simulink model "vehicle_hostmodel_2022b_Vignesh"  (R2022b)
settings: Solver=VariableStepAuto  StartTime=0  StopTime=1000  RelTol=1e-3
model workspace (MAT data in the model file):
  finalint = 0
  firstWarning = 1
  originalScenarioChecksum = '114339432DE22364D47BB28FC96DC10C'
undefined symbols (not defined in the file): Acceleration, ActorID, AngularVelocity, cameraParams, curvature, DefaultGear, DEND_B, DEND_S, DEND_T, direction, DiscIntNeverNeededParam, driving, gradbp, L, LF, LR, m, matlabshared, MAX_BRAKE, MAX_STEER, MAX_TORQUE, MCAR, MIN_BRAKE, MIN_STEER, MIN_TORQUE, n, NUMD_B, NUMD_S, NUMD_T, Pitch, Pose, Position, psi_o, R, Roll, RRdamp, SceneInfo, sigbuilder_block, STEER_RATIO, stopSign_ID, Tdead, thetaRefs, TL_ID, trackingParams, TrackWidth, Ts, ts, Vdead, Velocity, WB, X_o, xRef2s, Y_o, Yaw, yRef2, yRef2s
libraries: drivingscenarioandsensors x11, simulink x10, roadrunnerscenario x9, slrealtimeutilitieslib x7, slrealtimeiplib x7, simulink_extras x5, drivingvehiclecontroller x3, trackingutilitieslib x3, robotalgslib x2, slpidlib x2, drivinglib x2, eeGeneralControl x1
(part 4 of 5)

== system vehicle_hostmodel_2022b_Vignesh/Reference Data/Subsystem1/Subsystem2/Subsystem ==
  note: Select method to calculate theta
  Integrator : Inport
  Curvature : Lookup_n-D  NumberOfTableDimensions=1  BreakpointsForDimension1=gradbp  Table=curvature  InternalRulePriority=Speed  RndMeth=Simplest
  Direction : Lookup_n-D  NumberOfTableDimensions=1  BreakpointsForDimension1=gradbp  Table=direction  InternalRulePriority=Speed  RndMeth=Simplest
  From Workspace1 : FromWorkspace  VariableName=yRef2  SampleTime=-1
  From Workspace2 : FromWorkspace  VariableName=xRef2  SampleTime=-1
  From Workspace3 : FromWorkspace  VariableName=gradbp  SampleTime=-1
  Goto : Goto  Commented=on  GotoTag=xRef  TagVisibility=global
  Goto1 : Goto  Commented=on  GotoTag=yRef  TagVisibility=global
  Matrix Concatenate : Concatenate  Mode=Multidimensional array  ConcatenateDimension=2
  Mux : Mux  Inputs=3
  Switch Case : SwitchCase
  Theta : Subsystem  Variant=on  VariantControlMode=label  LabelModeActiveChoice=thetaLookUpTable
  X Ref : Lookup_n-D  NumberOfTableDimensions=1  BreakpointsForDimension1=gradbp  Table=xRef2s  InternalRulePriority=Speed  RndMeth=Simplest
  Y Ref : Lookup_n-D  NumberOfTableDimensions=1  BreakpointsForDimension1Source=Input port  BreakpointsForDimension1=gradbp  TableSource=Input port  Table=yRef2s  InternalRulePriority=Speed  RndMeth=Simplest
      settings: InputPortMap=u0,p221,p5
  Out1 : Outport
  Out2 : Outport  Port=2
  CurvatureO : Outport  Port=3
  DirectionO : Outport  Port=4
  finalint : Outport  Port=5
  wires:
  Direction/1 -> DirectionO/1
  Y Ref/1 -> Theta/1(y), Mux/2, Goto1/1
  Theta/1(theta) -> Mux/3
  X Ref/1 -> Theta/2(x), Mux/1, Goto/1
  Matrix Concatenate/1 -> Out1/1
  Curvature/1 -> CurvatureO/1
  Mux/1 -> Out2/1
  From Workspace1/1 -> Y Ref/2, Matrix Concatenate/2
  From Workspace2/1 -> Matrix Concatenate/1
  From Workspace3/1 -> Y Ref/3
  Integrator/1 -> Direction/1, Curvature/1, Theta/3(dis), Y Ref/1, X Ref/1

== system vehicle_hostmodel_2022b_Vignesh/Reference Data/Subsystem1/Subsystem3/Subsystem ==
  note: Select method to calculate theta
  xd : Inport
  yd : Inport  Port=2
  Integrator : Inport  Port=3
  Add Constant : Bias  Bias=6.5  SaturateOnIntegerOverflow=off
  Curvature : Lookup_n-D  NumberOfTableDimensions=1  BreakpointsForDimension1=gradbp  Table=curvature  InternalRulePriority=Speed  RndMeth=Simplest
  Direction : Lookup_n-D  NumberOfTableDimensions=1  BreakpointsForDimension1=gradbp  Table=direction  InternalRulePriority=Speed  RndMeth=Simplest
  From Workspace1 : FromWorkspace  VariableName=yRef2  SampleTime=-1
  From Workspace2 : FromWorkspace  VariableName=xRef2  SampleTime=-1
  From Workspace3 : FromWorkspace  VariableName=gradbp  SampleTime=-1
  Goto : Goto  Commented=on  GotoTag=xRef  TagVisibility=global
  Goto1 : Goto  Commented=on  GotoTag=yRef  TagVisibility=global
  Matrix Concatenate : Concatenate  Mode=Multidimensional array  ConcatenateDimension=2
  Mux : Mux  Inputs=3
  Theta : Subsystem  Variant=on  VariantControlMode=label  LabelModeActiveChoice=thetaLookUpTable
  X Ref : Lookup_n-D  NumberOfTableDimensions=1  BreakpointsForDimension1Source=Input port  BreakpointsForDimension1=gradbp  TableSource=Input port  Table=xRef2s  InternalRulePriority=Speed  RndMeth=Simplest
      settings: InputPortMap=u0,p221,p5
  Y Ref : Lookup_n-D  NumberOfTableDimensions=1  BreakpointsForDimension1Source=Input port  BreakpointsForDimension1=gradbp  TableSource=Input port  Table=yRef2s  InternalRulePriority=Speed  RndMeth=Simplest
      settings: InputPortMap=u0,p221,p5
  Out1 : Outport
  Out2 : Outport  Port=2
  CurvatureO : Outport  Port=3
  DirectionO : Outport  Port=4
  wires:
  Direction/1 -> DirectionO/1
  Theta/1(theta) -> Mux/3
  Matrix Concatenate/1 -> Out1/1
  Curvature/1 -> CurvatureO/1
  Mux/1 -> Out2/1
  From Workspace1/1 -> Add Constant/1, Matrix Concatenate/2
  From Workspace2/1 -> X Ref/2, Matrix Concatenate/1
  From Workspace3/1 -> Y Ref/3, X Ref/3
  X Ref/1 -> Theta/2(x), Mux/1
  Add Constant/1 -> Y Ref/2
  Y Ref/1 -> Theta/1(y), Mux/2
  Integrator/1 -> Direction/1, Curvature/1, Theta/3(dis), Y Ref/1, X Ref/1

== system vehicle_hostmodel_2022b_Vignesh/Reference Data/Subsystem2/Subsystem/Theta ==
  note: 1) Add Subsystem or Model blocks as valid variant choices.
      | 2) You cannot connect blocks at this level. At simulation, connectivity is automatically
      | determined, based on the active variant and port name matching.
  y : Inport
  x : Inport  Port=2
  dis : Inport  Port=3
  thetaBlocks : Subsystem  VariantControl=thetaSimulinkBlock
  thetaLt : Subsystem  VariantControl=thetaLookUpTable
  theta : Outport

== system vehicle_hostmodel_2022b_Vignesh/Reference Data/Subsystem3/Subsystem/Theta ==
  note: 1) Add Subsystem or Model blocks as valid variant choices.
      | 2) You cannot connect blocks at this level. At simulation, connectivity is automatically
      | determined, based on the active variant and port name matching.
  y : Inport
  x : Inport  Port=2
  dis : Inport  Port=3
  thetaBlocks : Subsystem  VariantControl=thetaSimulinkBlock
  thetaLt : Subsystem  VariantControl=thetaLookUpTable
  theta : Outport

== system vehicle_hostmodel_2022b_Vignesh/Roadrunner Port/Initiaal State/Initialize State/Calculate Initial States ==
  EgoRuntime : Inport
  Trigger : TriggerPort  VariantControl=(inherit)  InitialTriggerSignalState=negative  PortDimensions=1
  Calculate Initial States : MATLAB Function  TreatAsAtomicUnit=on
  EgoInitialState : Outport
  wires:
  EgoRuntime/1 -> Calculate Initial States/1(egoRuntime)
  Calculate Initial States/1(egoInitialState) -> EgoInitialState/1

== system vehicle_hostmodel_2022b_Vignesh/Roadrunner Port/Initiaal State/Pack Current States/Delayed Steering System ==
  SteerCmd : Inport
  Add : Sum  Inputs=+-
  Delay : TransferFcn  Denominator=[0.1 0]
  CurrSteer : Outport  VectorParamsAs1DForOutWhenUnconnected=off
  wires:
  Add/1 -> Delay/1
  SteerCmd/1 -> Add/1
  Delay/1 -> CurrSteer/1, Add/2

== system vehicle_hostmodel_2022b_Vignesh/Controllers/Subsystem3/Subsystem1/Subsystem2/Subsystem ==
  acc_cmd : Inport
  Constant1 : Constant  Value=MCAR
  Gain : Gain  Gain=1.1*MCAR
  Gain1 : Gain  Gain=1.2*0.3*2/2
  Gain2 : Gain  Gain=0.7*9.81
  Gain4 : Gain  Gain=R/(7.05*0.8)
  Integrator : Integrator  ExternalReset=falling
  Square : Math  Operator=square
  Sum : Sum  Inputs=+++
  T_eng_cmd : Outport
  wires:
  Constant1/1 -> Gain2/1
  Gain/1 -> Sum/3
  Sum/1 -> Gain4/1
  acc_cmd/1 -> Gain/1, Integrator/2, Integrator/1
  Gain2/1 -> Sum/2
  Gain1/1 -> Sum/1  "F_aero"
  Gain4/1 -> T_eng_cmd/1  "T_eng"
  Integrator/1 -> Square/1  "v"
  Square/1 -> Gain1/1

== system vehicle_hostmodel_2022b_Vignesh/Controllers/Subsystem3/Subsystem1/Subsystem2/Subsystem1 ==
  decc_cmd : Inport
  Constant1 : Constant  Value=MCAR
  Gain : Gain  Gain=1.1*MCAR
  Gain1 : Gain  Gain=1.2*0.3*2/2
  Gain2 : Gain  Gain=0.7*9.81
  Gain4 : Gain  Gain=-R/(7.05*0.8)
  Integrator : Integrator  ExternalReset=falling
  Square : Math  Operator=square
  Sum : Sum  Inputs=+++
  T_brake_cmd : Outport
  wires:
  Square/1 -> Gain1/1
  Integrator/1 -> Square/1  "v"
  Gain4/1 -> T_brake_cmd/1  "T_eng"
  Gain1/1 -> Sum/1  "F_aero"
  Gain2/1 -> Sum/2
  decc_cmd/1 -> Integrator/2, Integrator/1, Gain/1
  Sum/1 -> Gain4/1
  Gain/1 -> Sum/3
  Constant1/1 -> Gain2/1

== system vehicle_hostmodel_2022b_Vignesh/Controllers/Subsystem3/Subsystem2/Subsystem2/Subsystem ==
  acc_cmd : Inport
  Constant1 : Constant  Value=MCAR
  Gain : Gain  Gain=1.1*MCAR
  Gain1 : Gain  Gain=1.2*0.3*2/2
  Gain2 : Gain  Gain=0.7*9.81
  Gain4 : Gain  Gain=R/(7.05*0.8)
  Integrator : Integrator  ExternalReset=falling
  Square : Math  Operator=square
  Sum : Sum  Inputs=+++
  T_eng_cmd : Outport
  wires:
  Constant1/1 -> Gain2/1
  Gain/1 -> Sum/3
  Sum/1 -> Gain4/1
  acc_cmd/1 -> Gain/1, Integrator/2, Integrator/1
  Gain2/1 -> Sum/2
  Gain1/1 -> Sum/1  "F_aero"
  Gain4/1 -> T_eng_cmd/1  "T_eng"
  Integrator/1 -> Square/1  "v"
  Square/1 -> Gain1/1

== system vehicle_hostmodel_2022b_Vignesh/Controllers/Subsystem3/Subsystem2/Subsystem2/Subsystem1 ==
  decc_cmd : Inport
  Constant1 : Constant  Value=MCAR
  Gain : Gain  Gain=1.1*MCAR
  Gain1 : Gain  Gain=1.2*0.3*2/2
  Gain2 : Gain  Gain=0.7*9.81
  Gain4 : Gain  Gain=-R/(7.05*0.8)
  Integrator : Integrator  ExternalReset=falling
  Square : Math  Operator=square
  Sum : Sum  Inputs=+++
  T_brake_cmd : Outport
  wires:
  Square/1 -> Gain1/1
  Integrator/1 -> Square/1  "v"
  Gain4/1 -> T_brake_cmd/1  "T_eng"
  Gain1/1 -> Sum/1  "F_aero"
  Gain2/1 -> Sum/2
  decc_cmd/1 -> Integrator/2, Integrator/1, Gain/1
  Sum/1 -> Gain4/1
  Gain/1 -> Sum/3
  Constant1/1 -> Gain2/1

== system vehicle_hostmodel_2022b_Vignesh/Reference Data/Subsystem1/Subsystem2/Subsystem/Theta ==
  note: 1) Add Subsystem or Model blocks as valid variant choices.
      | 2) You cannot connect blocks at this level. At simulation, connectivity is automatically
      | determined, based on the active variant and port name matching.
  y : Inport
  x : Inport  Port=2
  dis : Inport  Port=3
  thetaBlocks : Subsystem  VariantControl=thetaSimulinkBlock
  thetaLt : Subsystem  VariantControl=thetaLookUpTable
  theta : Outport

== system vehicle_hostmodel_2022b_Vignesh/Reference Data/Subsystem1/Subsystem3/Subsystem/Theta ==
  note: 1) Add Subsystem or Model blocks as valid variant choices.
      | 2) You cannot connect blocks at this level. At simulation, connectivity is automatically
      | determined, based on the active variant and port name matching.
  y : Inport
  x : Inport  Port=2
  dis : Inport  Port=3
  thetaBlocks : Subsystem  VariantControl=thetaSimulinkBlock
  thetaLt : Subsystem  VariantControl=thetaLookUpTable
  theta : Outport

== system vehicle_hostmodel_2022b_Vignesh/Reference Data/Subsystem2/Subsystem/Theta/thetaBlocks ==
  note: theta calculated from Simulink blocks
  y : Inport
  x : Inport  Port=2
  dis : Inport  Port=3
  Atan2 : Trigonometry  Operator=atan2  ApproximationMethod=CORDIC
  Difference : simulink/Discrete/Difference  ICPrevInput=0.0  OutMin=[]  OutMax=[]  OutDataType=fixdt(1, 16)  OutScaling=2^-10  DoSatur=off
  Difference1 : simulink/Discrete/Difference  ICPrevInput=0.0  OutMin=[]  OutMax=[]  OutDataType=fixdt(1, 16)  OutScaling=2^-10  DoSatur=off
  IC : InitialCondition  Value=psi_o
  Radians to Degrees : simulink_extras/Transformations/Radians to Degrees
  Terminator : Terminator
  theta : Outport
  wires:
  IC/1 -> Radians to Degrees/1
  Atan2/1 -> IC/1
  dis/1 -> Terminator/1
  x/1 -> Difference1/1
  y/1 -> Difference/1
  Radians to Degrees/1 -> theta/1
  Difference/1 -> Atan2/1
  Difference1/1 -> Atan2/2

== system vehicle_hostmodel_2022b_Vignesh/Reference Data/Subsystem2/Subsystem/Theta/thetaLt ==
  note: Check out the script "setUpModel" to understand how we have calculated theta
  note: theta based on lookup table
  y : Inport
  x : Inport  Port=2
  dis : Inport  Port=3
  Terminator : Terminator
  Terminator1 : Terminator
  Theta Ref : Lookup_n-D  NumberOfTableDimensions=1  BreakpointsForDimension1=gradbp  Table=thetaRefs  InternalRulePriority=Speed  RndMeth=Simplest
  theta : Outport
  wires:
  Theta Ref/1 -> theta/1
  dis/1 -> Theta Ref/1
  x/1 -> Terminator1/1
  y/1 -> Terminator/1

== system vehicle_hostmodel_2022b_Vignesh/Reference Data/Subsystem3/Subsystem/Theta/thetaBlocks ==
  note: theta calculated from Simulink blocks
  y : Inport
  x : Inport  Port=2
  dis : Inport  Port=3
  Atan2 : Trigonometry  Operator=atan2  ApproximationMethod=CORDIC
  Difference : simulink/Discrete/Difference  ICPrevInput=0.0  OutMin=[]  OutMax=[]  OutDataType=fixdt(1, 16)  OutScaling=2^-10  DoSatur=off
  Difference1 : simulink/Discrete/Difference  ICPrevInput=0.0  OutMin=[]  OutMax=[]  OutDataType=fixdt(1, 16)  OutScaling=2^-10  DoSatur=off
  IC : InitialCondition  Value=psi_o
  Radians to Degrees : simulink_extras/Transformations/Radians to Degrees
  Terminator : Terminator
  theta : Outport
  wires:
  IC/1 -> Radians to Degrees/1
  Atan2/1 -> IC/1
  dis/1 -> Terminator/1
  x/1 -> Difference1/1
  y/1 -> Difference/1
  Radians to Degrees/1 -> theta/1
  Difference/1 -> Atan2/1
  Difference1/1 -> Atan2/2

== system vehicle_hostmodel_2022b_Vignesh/Reference Data/Subsystem3/Subsystem/Theta/thetaLt ==
  note: Check out the script "setUpModel" to understand how we have calculated theta
  note: theta based on lookup table
  y : Inport
  x : Inport  Port=2
  dis : Inport  Port=3
  Terminator : Terminator
  Terminator1 : Terminator
  Theta Ref : Lookup_n-D  NumberOfTableDimensions=1  BreakpointsForDimension1=gradbp  Table=thetaRefs  InternalRulePriority=Speed  RndMeth=Simplest
  theta : Outport
  wires:
  Theta Ref/1 -> theta/1
  dis/1 -> Theta Ref/1
  x/1 -> Terminator1/1
  y/1 -> Terminator/1

== system vehicle_hostmodel_2022b_Vignesh/Reference Data/Subsystem1/Subsystem2/Subsystem/Theta/thetaBlocks ==
  note: theta calculated from Simulink blocks
  y : Inport
  x : Inport  Port=2
  dis : Inport  Port=3
  Atan2 : Trigonometry  Operator=atan2  ApproximationMethod=CORDIC
  Difference : simulink/Discrete/Difference  ICPrevInput=0.0  OutMin=[]  OutMax=[]  OutDataType=fixdt(1, 16)  OutScaling=2^-10  DoSatur=off
  Difference1 : simulink/Discrete/Difference  ICPrevInput=0.0  OutMin=[]  OutMax=[]  OutDataType=fixdt(1, 16)  OutScaling=2^-10  DoSatur=off
  IC : InitialCondition  Value=psi_o
  Radians to Degrees : simulink_extras/Transformations/Radians to Degrees
  Terminator : Terminator
  theta : Outport
  wires:
  IC/1 -> Radians to Degrees/1
  Atan2/1 -> IC/1
  dis/1 -> Terminator/1
  x/1 -> Difference1/1
  y/1 -> Difference/1
  Radians to Degrees/1 -> theta/1
  Difference/1 -> Atan2/1
  Difference1/1 -> Atan2/2

== system vehicle_hostmodel_2022b_Vignesh/Reference Data/Subsystem1/Subsystem2/Subsystem/Theta/thetaLt ==
  note: Check out the script "setUpModel" to understand how we have calculated theta
  note: theta based on lookup table
  y : Inport
  x : Inport  Port=2
  dis : Inport  Port=3
  Terminator : Terminator
  Terminator1 : Terminator
  Theta Ref : Lookup_n-D  NumberOfTableDimensions=1  BreakpointsForDimension1=gradbp  Table=thetaRefs  InternalRulePriority=Speed  RndMeth=Simplest
  theta : Outport
  wires:
  Theta Ref/1 -> theta/1
  dis/1 -> Theta Ref/1
  x/1 -> Terminator1/1
  y/1 -> Terminator/1

== system vehicle_hostmodel_2022b_Vignesh/Reference Data/Subsystem1/Subsystem3/Subsystem/Theta/thetaBlocks ==
  note: theta calculated from Simulink blocks
  y : Inport
  x : Inport  Port=2
  dis : Inport  Port=3
  Atan2 : Trigonometry  Operator=atan2  ApproximationMethod=CORDIC
  Difference : simulink/Discrete/Difference  ICPrevInput=0.0  OutMin=[]  OutMax=[]  OutDataType=fixdt(1, 16)  OutScaling=2^-10  DoSatur=off
  Difference1 : simulink/Discrete/Difference  ICPrevInput=0.0  OutMin=[]  OutMax=[]  OutDataType=fixdt(1, 16)  OutScaling=2^-10  DoSatur=off
  IC : InitialCondition  Value=psi_o
  Radians to Degrees : simulink_extras/Transformations/Radians to Degrees
  Terminator : Terminator
  theta : Outport
  wires:
  IC/1 -> Radians to Degrees/1
  Atan2/1 -> IC/1
  dis/1 -> Terminator/1
  x/1 -> Difference1/1
  y/1 -> Difference/1
  Radians to Degrees/1 -> theta/1
  Difference/1 -> Atan2/1
  Difference1/1 -> Atan2/2

== system vehicle_hostmodel_2022b_Vignesh/Reference Data/Subsystem1/Subsystem3/Subsystem/Theta/thetaLt ==
  note: Check out the script "setUpModel" to understand how we have calculated theta
  note: theta based on lookup table
  y : Inport
  x : Inport  Port=2
  dis : Inport  Port=3
  Terminator : Terminator
  Terminator1 : Terminator
  Theta Ref : Lookup_n-D  NumberOfTableDimensions=1  BreakpointsForDimension1=gradbp  Table=thetaRefs  InternalRulePriority=Speed  RndMeth=Simplest
  theta : Outport
  wires:
  Theta Ref/1 -> theta/1
  dis/1 -> Theta Ref/1
  x/1 -> Terminator1/1
  y/1 -> Terminator/1

== matlab function vehicle_hostmodel_2022b_Vignesh/Environment & Data/Visualisation & Data/Positions and States /MATLAB Function2 ==
  data: Actors input; ss_poses output; ss_State input

function ss_poses = findssposes(Actors, ss_State)

n=length(ss_State);
ss_poses=zeros(n,4);
indices=zeros(n,1);
ID=zeros(length(Actors),1);

for i=1:length(Actors)
 ID(i)=Actors(i).ActorID;
end

indices=find(ismember(ID,ss_State));
if(~isempty(indices))
    
    for i=1:n
        ss_poses(i,:)=([Actors(indices(i)).Position(:)',ss_State(i)]);
    end
end

ss_poses(ss_poses==0)=NaN;






% ss1_poses=zeros(1,4);
% ss2_poses=zeros(1,4);
% for i=1:length(Actors)
%     ID=Actors(i).ActorID;
%     
%     if(ID==ss1_State(1))
%         ss1_poses=[Actors(i).Position(:)',ss1_State(1)];
%     elseif ID== (ss1_State(2))
%         ss2_poses=[Actors(i).Position(:)',ss1_State(2)];
%     
%     end
%   
% end
% ss1_poses(ss1_poses==0)=NaN;   
% ss2_poses(ss2_poses==0)=NaN;

== matlab function vehicle_hostmodel_2022b_Vignesh/Environment & Data/Visualisation & Data/Positions and States /MATLAB Function1 ==
  data: Actors input; TL_poses output; TL_State input

function TL_poses = findTLposes(Actors, TL_State)
n=length(TL_State);
TL_poses=zeros(n/2,5);
indices=zeros(n/2,1);
ID=zeros(length(Actors),1);

for i=1:length(Actors)
 ID(i)=Actors(i).ActorID;
end

indices=find(ismember(ID,TL_State(n/2+1:end)));
if (~isempty(indices))

    for i=1:n/2
        TL_poses(i,:)=([Actors(indices(i)).Position(:)',TL_State(i),ID(indices(i))]);

    end
end
TL_poses(TL_poses==0)=NaN;

== stateflow chart vehicle_hostmodel_2022b_Vignesh/Environment & Data/Visualisation & Data/Positions and States /Traffic Light Sensor/Traffic Light Switching Logic ==
  state STEADYRED
    entry:
    trafficLight(:)= Red; TL_ID=TL_id;
  state STEADYGREEN
    entry:
    trafficLight(:)= Green; TL_ID=TL_id;
  state START
    entry:
    trafficLight=TL_id;
    trafficLight(:)= Black;TL_ID=TL_id;
  state TRAFFICLIGHT_ODDYELLOW_EVENRED
    entry:
    trafficLight(1:2:end)=Yellow;TL_ID(1:2:end)=TL_id(1:2:end);
    trafficLight(2:2:end) = Red;TL_ID(2:2:end)=TL_id(2:2:end);
  state TRAFFICLIGHT_ODDGREEN_EVENRED
    entry:
    trafficLight(1:2:end)=Green;TL_ID(1:2:end)=TL_id(1:2:end);
    trafficLight(2:2:end) = Red;TL_ID(2:2:end)=TL_id(2:2:end);
  state TRAFFICLIGHT_ODDRED_EVENYELLOW
    entry:
    trafficLight(1:2:end)=Red;TL_ID(1:2:end)=TL_id(1:2:end);
    trafficLight(2:2:end) = Yellow;TL_ID(2:2:end)=TL_id(2:2:end);
  state TRAFFICLIGHT_ODDRED_EVENGREEN
    entry:
    trafficLight(1:2:end)=Red;TL_ID(1:2:end)=TL_id(1:2:end);
    trafficLight(2:2:end) = Green;TL_ID(2:2:end)=TL_id(2:2:end);
  (default) -> START
  START -> STEADYGREEN [order 3] : [LightConfig==1]
  START -> STEADYRED [order 1] : [LightConfig==2]
  START -> TRAFFICLIGHT_ODDGREEN_EVENRED [order 2] : [LightConfig ==3]
  TRAFFICLIGHT_ODDGREEN_EVENRED -> TRAFFICLIGHT_ODDYELLOW_EVENRED : after(4,sec)
  TRAFFICLIGHT_ODDYELLOW_EVENRED -> TRAFFICLIGHT_ODDRED_EVENGREEN : after(1,sec)
  TRAFFICLIGHT_ODDRED_EVENYELLOW -> TRAFFICLIGHT_ODDGREEN_EVENRED : after(1,sec)
  TRAFFICLIGHT_ODDRED_EVENGREEN -> TRAFFICLIGHT_ODDRED_EVENYELLOW : after(4,sec)
  data: Green constant double =3; Red constant double =1; Yellow constant double =2; LightConfig input; TL_id input; Black constant double =0; TL_ID output; trafficLight output

== matlab function vehicle_hostmodel_2022b_Vignesh/Environment & Data/Sensors & Perception/MATLAB Function ==
  data: SceneID output; ObjRelVel output; SceneRelVel output; SceneDist output; ObjectDist output; ObjAhead output; SDist input; Tracking input; SceneAhead output; RelVelmin output; RelDistmin output; Trans input; ObjectMIO_Position output
function [SceneID,ObjRelVel,SceneRelVel,SceneDist,ObjectDist,ObjAhead,SceneAhead,RelVelmin,RelDistmin,ObjectMIO_Position]= SFDetections(SDist,Tracking, Trans)
ObjectID = zeros(20,1);
TrackPos = zeros(3,20);
TrackVel = zeros(3,20);
ObjectDist = 100; % zeros(20,1);
SceneDist = 100;
ObjRelVel = 10;
SceneRelVel = 10;
% ScenePos = [0 0];
ObjAhead = 0;
SceneAhead = 0;
SceneID = 0;
TracksNum = Tracking.NumTracks;
ObjectMIO_Position = zeros(3,1);


for t = 1:TracksNum
    ObjectID(t) = Tracking.Tracks(t).ObjectClassID;
    TrackPos(:,t) = Tracking.Tracks(t).State(1:2:5);
    TrackVel(:,t) = Tracking.Tracks(t).State(2:2:6);
   
    if TrackPos(2,t) < 1 && TrackPos(2,t) > -4 && abs(TrackPos(1,t)) <= SDist
        
        if ObjectID(t) >= 7 % 7=SS 8=TL 9=RA 10=RRC % labels {1,2,3,4} => {'TrafficLight','StopSign','RailRoadCrossing','RoundAbout'};
            SceneAhead = 1;
            SceneDist = min(SceneDist,TrackPos(1,t));
            if TrackPos(1,t) <= SceneDist
                % ScenePos = TrackPos(1:2,t)';
                SceneRelVel = TrackVel(1,t);
                SceneID = ObjectID(t);
            end
        end

        if ObjectID(t) < 7 && ObjectID(t) > 0
            ObjAhead = 1;
            ObjectDist = min(ObjectDist,TrackPos(1,t));
            ObjectMIO_Position(:,1) = TrackPos(:,t);

            if TrackPos(1,t) <= ObjectDist
                ObjRelVel = TrackVel(1,t);
                ObjID = ObjectID(t);
            end
        end

    end
    
end

if Trans == 1  % ObjectDist <= SceneDist
    RelVelmin = ObjRelVel;
    RelDistmin = ObjectDist;
else
    RelVelmin = min(SceneRelVel,ObjRelVel);
    RelDistmin = min(SceneDist,ObjectDist);
end

== matlab function vehicle_hostmodel_2022b_Vignesh/Vehicle Dynamics/Info2ActorState/MATLAB Function ==
  data: X input; Position output; Y input; Z input
function Position = fcn(X, Y, Z)

Position = [X Y, Z];

== matlab function vehicle_hostmodel_2022b_Vignesh/Subsystem/PathPlanner/MATLAB Function4 ==
  data: Distance output; output input; CurrentPose input; point output
function [Distance,point] = d2f(output,CurrentPose)



%Distance = norm(output(end,:) - CurrentPose(1:2)');
Distance= output(end,1)- CurrentPose(1);
point=output(end,:);

end

%Distance = sqrt(CurrentPose(1)-output(99,1))^2 + (CurrentPose(2)-output(99,2)^2);
%CurrentPose
%output=zeros(99,2);
%lastPoint = output(end,:);
%dx = lastPoint(1) - x;
%dx= output(end,1)-x;
%dy = output(end,2) - y;
%distance = sqrt(dx^2 + dy^2);

== matlab function vehicle_hostmodel_2022b_Vignesh/Environment & Data/Sensors & Perception/MATLAB Function1 ==
  data: EVpos input; yaw input; SceneID input; SceneInfo input; SDir output; SDist input; D2S output
function [SDir,D2S] = SceneFinder(EVpos,yaw, SceneID, SceneInfo, SDist)
D2S = zeros(10,1);
    % dist = zeros(1,length(SceneLocations));
    for j = 1:length(SceneInfo(:,1))
        distXY = SceneInfo(j,1:2) - EVpos(1:2);
        D2S(j) = norm(distXY);
        
%         if (D2S <= SDist)
%             Scene = SceneInfo(j,3); % labels {1,2,3,4} => {'TrafficLight','StopSign','RailRoadCrossing','RoundAbout'};
%             angl = atan2d(distXY(2),distXY(1));
%             angl = angl - yaw;
% %             rot = [cosd(angl) -sind(angl);sind(angl) cosd(angl)];
% %             distXY = rot*distXY';
% %             angl = atan2d(distXY(2),distXY(1));
%             
%             if angl < 0
%                 angl = angl + 360;
%             end
% 
%             if (angl > 315) || (angl <= 45) 
%                 SDir = "N";
%             elseif (angl > 225) && (angl <= 315)
%                 SDir = "E";
%             elseif (angl > 135) && (angl <= 225)
%                 SDir = "S";
%                 D2S = 1000;
%                 angl = 1000;
%                 Scene = 0;
%             elseif (angl > 45) && (angl <= 135)
%                 SDir = "W";
%             else
%                 SDir = "Error";
%             end
%             break
%         else
%             Scene = 0;
%             SDir = " ";
%             angl = 1000;
%             D2S = 1000;
%         end

    end
[val,indx] = min(D2S);

== matlab function vehicle_hostmodel_2022b_Vignesh/Subsystem/Function-Call Subsystem/MATLAB Function2 ==
  data: EgoPosition input; MIOPos input; curvature input; MIOVel input; V_i input; xd output; yd output; laneL input; laneR input; V_desired input; LCinProgress output
function [xd,yd,LCinProgress] = traj(EgoPosition,MIOPos,curvature,MIOVel, V_i, laneL, laneR, V_desired)
Vx_i =0;Vx_f=0;Vy_i=0;Vy_f=0;Ax_i=0;Ax_f=0;Ay_i=0;Ay_f=0;T_i=0;T_f=0;V_f=0;A_f=0;x_set=0;y_set=0;theta4=0;

P = zeros(6,6);
% xq = zeros(1,size(RefPath,1)); yq = zeros(1,size(RefPath,2));
EgoPosition(1,2)=-EgoPosition(1,2)
x_init= EgoPosition(1,1)+0.5; y_init = EgoPosition(1,2)-0.8;
% xq = RefPath(:,1)'; 
% yq = RefPath(:,2)';
num_foc_t = 98;
V_max= V_desired; ad_n=0; vd_n=MIOVel; wd_n=vd_n*curvature;
lane_width = 3.6 * (laneL-laneR); % +1 if left of current lane and -1 if right of current lane
xd = zeros(num_foc_t+1,1); 
yd = zeros(num_foc_t+1,1);
xf =0; 
yf = 0;

    %xf = [EgoPosition(1,1)+ MIOPos(1) ]; yf = [ EgoPosition(1,2)+ MIOPos(2) + lane_width];  
    xf = [EgoPosition(1,1)+ 40 ]; yf = [ EgoPosition(1,2)+ 1.1*lane_width]; % 80
    V_f = V_max;
    W_f = V_f*curvature;
    A_f = 0;

    %dist2crash = sqrt((x_init-MIOPos(1))^2+(y_init-MIOPos(2))^2);
    %dist2crash = 40;
    %T_f = abs(dist2crash/(MIOVel-V_i));
    T_f = 3;
    P = [1, T_i, T_i^2, T_i^3, T_i^4, T_i^5;
         0, 1, 2*T_i, 3*T_i^2, 4*T_i^3, 5*T_i^4;
         0, 0, 2, 6*T_i, 12*T_i^2, 20*T_i^3;
         1, T_f, T_f^2, T_f^3, T_f^4, T_f^5;
         0, 1, 2*T_f, 3*T_f^2, 4*T_f^3, 5*T_f^4;
         0, 0, 2, 6*T_f, 12*T_f^2, 20*T_f^3];

%     mtang4 = (yq(1,index+2)-yq(1,index+1))/(xq(1,index+2)-xq(1,index+1));

    Vx_i = vd_n*cos(theta4); 
    Vy_i = vd_n*sin(theta4); 
    Ax_i = ad_n*cos(theta4)-vd_n*sin(theta4)*wd_n; 
    Ay_i = ad_n*sin(theta4)+vd_n*cos(theta4)*wd_n;

%     if(xq(index+2)-xq(index+1)<0)
%         theta_4 = pi + atan(mtang4);
%     else
%         theta_4 = atan(mtang4);
%     end

    theta_4 =0;
    Vx_f = V_f*cos(theta_4); % curvature angle
    Vy_f = V_f*sin(theta_4);
    Ax_f = A_f*cos(theta_4)-V_f*sin(theta_4)*W_f;
    Ay_f = A_f*sin(theta_4)+V_f*cos(theta_4)*W_f;

    g1 = [x_init; Vx_i; Ax_i; xf; Vx_f; Ax_f];
    g2 = [y_init; Vy_i; Ay_i; yf; Vy_f; Ay_f];

    a_coeff = P\g1;
    b_coeff = P\g2;
    
    td = T_i;
    scatter(x_init,y_init,'go')
    hold on; 
    scatter(xf,yf,'ro')
    hold on;
    
    for f = 1:(num_foc_t+1)
        xd(f,1) = [1,td,td^2,td^3,td^4,td^5]*a_coeff 
        yd(f,1) = [1,td,td^2,td^3,td^4,td^5]*b_coeff
        td = td + (T_f - T_i)/num_foc_t;
        scatter(xd(f,1),yd(f,1),'y.');
    end

LCinProgress = 1;

% hold on;
end

== matlab function vehicle_hostmodel_2022b_Vignesh/Roadrunner Port/Initiaal State/Initialize State/Calculate Initial States/Calculate Initial States ==
  data: egoRuntime input; egoInitialState output Bus: BusVehicleInfo
function egoInitialState = getInitialState(egoRuntime)
%getInitialState calculates initial conditions of the vehicle

% Calculate velocity
velocity = norm(egoRuntime.ActorRuntime.Velocity,2);
% Get Transformation matrix
transformationMatrix = egoRuntime.ActorRuntime.Pose;
% Get pose information
x = transformationMatrix(1,4);
y = transformationMatrix(2,4);
yaw = atan2d(-transformationMatrix(1,2), ...
            transformationMatrix(1,1));
% Pack the initial states
egoInitialState = struct('CurrPose', [y, -x, yaw], ...
    'CurrVelocity', velocity, ...
    'CurrYawRate', 0, ...
    'CurrSteer',0, ...
    'Direction',1);

== matlab function vehicle_hostmodel_2022b_Vignesh/Controllers/Subsystem3/Subsystem2/MATLAB Function ==
  data: u input; accel output; decel output
function [accel, decel] = fcn(u)
if(u>0)
    accel=u; decel=0;
elseif(u<0)
    accel=0; decel=-u;
else
    accel=0;decel=0;
end

== matlab function vehicle_hostmodel_2022b_Vignesh/Controllers/MATLAB Function2 ==
  data: v input; RefVelCmd output; curvature input
function RefVelCmd = fcn(v,curvature)

    if abs(curvature) >= 0 && abs(curvature) <= 1e-2
        RefVelCmd = v;
    else
        r = 1/abs(curvature);
        RefVelCmd = min(v,sqrt(9.81*r*.2));
    end

== matlab function vehicle_hostmodel_2022b_Vignesh/Vehicle Dynamics/Info2ActorState/MATLAB Function1 ==
  data: Xdot input; Velocity output; Ydot input; Zdot input
function Velocity = fcn(Xdot, Ydot, Zdot)

Velocity = [Xdot Ydot, Zdot];

== matlab function vehicle_hostmodel_2022b_Vignesh/Roadrunner Port/MATLAB Function ==
  data: ActorsIn input; EgoVeh input; EgoRefActors output Bus: BusWorldToVehicleActors
function EgoRefActors  = GlobaltoEgoRefConv(ActorsIn,EgoVeh)
%ActorsOut = Simulink.Bus;
ActorsOut = ActorsIn;
numActors = length(ActorsIn.Actors);
for k = 1:numActors
    actorOut = driving.scenario.targetsToEgo(ActorsIn.Actors(k),EgoVeh);
    ActorsOut.Actors(k).ActorID             = actorOut.ActorID;
    ActorsOut.Actors(k).Position            = actorOut.Position;
    ActorsOut.Actors(k).Velocity            = actorOut.Velocity;
    ActorsOut.Actors(k).Roll                = actorOut.Roll;
    ActorsOut.Actors(k).Pitch               = actorOut.Pitch;
    ActorsOut.Actors(k).Yaw                 = actorOut.Yaw;
    ActorsOut.Actors(k).AngularVelocity    = actorOut.AngularVelocity;
end
EgoRefActors = ActorsOut;
end

== matlab function vehicle_hostmodel_2022b_Vignesh/MATLAB Function ==
  data: ttc output; dist output; left output; right output; LL_avail output; RL_avail output; tend2stay output; ego input; act input; LaneBounds input; RoadSpeed input; ego_vel output; stay output; LL_Change output; RL_Change output; y_lane output; LCinProgress input
function [ttc,dist,left,right,LL_avail,RL_avail,tend2stay,ego_vel,stay,LL_Change,RL_Change,y_lane] = fcn(ego,act,LaneBounds,RoadSpeed, LCinProgress)                       


%% Major tasks to look into

% Check the performance while transitioning into another lane 
% Lane change output when the ego on extreme lanes.
% Develop code to handle lane changes on road curvatures
% Integrate with the trajectory generation and check the perfomance
% Convert the code to ego vehicle coordinates


%%
%define some parameters
r_c = 20; %range considered to MIOs
t_min =  2;

num_actors = length(act.Actors);
%num_lanes = length(LaneBounds.LaneBoundaries)-1;


%% Using sensor data 
% TracksNum = Tracking.NumTracks;
% 
% 
% for t = 1:TracksNum
%     ObjectID(t) = Tracking.Tracks(t).ObjectClassID;
%     TrackPos(:,t) = Tracking.Tracks(t).State(1:2:5);
%     TrackVel(:,t) = Tracking.Tracks(t).State(2:2:6);

%% ego position and  velocity magnitude
ego_pos = ego.Position;
ego_vel = ego.Velocity(1);  % velocity

%ttc: (array) : agent.relative position / abs(relative velocity)
ttc = zeros(1,num_actors);
left = zeros(1,num_actors);
right = zeros(1,num_actors);

dist =  zeros(1,num_actors);
tend2stay=1;

%%
y_lane = zeros(1,length(LaneBounds.LaneBoundaries))

for l=1:length(y_lane)
    y_lane(l)=LaneBounds.LaneBoundaries(l).Coordinates(end,2)
end

%%
for i= 1:num_actors

    % Grab actor positions and velocities
    actor_pos = act.Actors(i).Position;   
    actor_vel = act.Actors(i).Velocity(1);  % x-component velocity

    %relative velocity of the agent
    rel_vel = actor_vel - ego_vel;


    %% Check if the actor is within a r_c range. If it is out of range, pass lane change as '1' automatically.

   dist(i) = norm([actor_pos(1) actor_pos(2)]-[ego_pos(1) ego_pos(2)]);
        
    if dist(i) > r_c
        left(i)=1;
        right(i)=1;
        continue
    end

    %% Check if the actor is in the same lane as that of ego

    % If the actor and ego are in the same lane, it is considered a lead/following vehicle in the same lane and by defualt, the lane change flag is 1.

    if (actor_pos(2)< (ego_pos(2)+0.5) && actor_pos(2) > (ego_pos(2)-0.5))
        if (rel_vel < 0 && ego_vel < (RoadSpeed+5) && actor_pos(1) > ego_pos(1) )
            left(i) =1;
            right(i)=1;
            tend2stay=0;        % we need to incorporate too slow condition even when the relative velocity is greater than 0.

        elseif (rel_vel < 0 && ego_vel < (RoadSpeed+5) && actor_pos(1) < ego_pos(1) )
            left(i) =1;
            right(i)=1;
            tend2stay=1;
        end

        continue
    end

    
    %% calculate ttc for the rest of the vehicles


    ttc(i) = (actor_pos(1)-ego_pos(1))/abs(rel_vel);

    % checking conditions for other surrounding actors

    % all actors on the left lane of the ego vehicle
%%
    if actor_pos(2)-ego_pos(2) > 0  

        if and(rel_vel>0, ttc(i) > t_min)  % target vehicles on the front of ego vehicle (any lane)
    
            left(i)=1; 
            right(i)=1;
    
        elseif (ttc(i)<0 && rel_vel<0 && abs(ttc(i)) > t_min)    % target vehicle on the back of ego vehicle (ttc<0) (any lane)
            left(i) =1;
            right(i)=1;
    
        else 
            left(i) =0;
            right(i)=1;
    
        end

    % all actors on the right lane of the ego vehicle

    elseif actor_pos(2)-ego_pos(2) < 0
         
        if and(rel_vel>0, ttc(i) > t_min)  % target vehicles on the front of ego vehicle (any lane)
    
            left(i)=1;
            right(i)=1;
    
        elseif (ttc(i)<0 && rel_vel<0 && abs(ttc(i)) > t_min)    % target vehicle on the back of ego vehicle (ttc<0) (any lane)
            left(i) =1;
            right(i)=1;
    
        else 
            left(i) =1;
            right(i)=0;
    
        end
    end
%%

end

%% check if the vehicle is in the extreme end lanes

    if ego_pos(2)<y_lane(1) && ego_pos(2)>y_lane(2)

        LL=0; RL=1;
    elseif ego_pos(2) > y_lane(end) && ego_pos(2) < y_lane(end-1)
        RL=0; LL=1;
    else 

        RL=1;LL=1;
    end

%%
LL_avail = all(left) %&& LL;

RL_avail = all(right) %&& RL               %&& ~lcLeft ; this can be decided later 


%% final commands

stay = tend2stay || ~(tend2stay || LL_avail || RL_avail);
LL_Change =  ~tend2stay && LL_avail ;

RL_Change =  ~tend2stay && RL_avail && ~LL_Change ;
LCFlag = ~stay;
if LCFlag && LCinProgress
    LCFlag = false;
    stay = ~LCFlag;
end

%% 






end

== matlab function vehicle_hostmodel_2022b_Vignesh/Vehicle Dynamics/Info2ActorState/MATLAB Function2 ==
  data: aX input; Acceleration output; aY input; aZ input
function Acceleration = fcn(aX, aY, aZ)

Acceleration = [aX aY, aZ];

== matlab function vehicle_hostmodel_2022b_Vignesh/Vehicle Dynamics/Info2ActorState/MATLAB Function3 ==
  data: phiDot input; AngularVelocity output; thetaDot input; psiDot input
function AngularVelocity = fcn(phiDot, thetaDot, psiDot)

AngularVelocity = [phiDot thetaDot, psiDot];

== stateflow chart vehicle_hostmodel_2022b_Vignesh/Vehicle Dynamics/VehicleDynamics/engine-steer-brake dynamics/GearSelection1 ==
  state Park
    CurrGear = 0;
  state Reverse
    CurrGear = -1;
  state drive
    CurrGear = 1;
  (default) -> (junction 12)
  (junction 12) -> Reverse [order 3] : [DefaultGear == -1]
  (junction 12) -> drive [order 2] : [DefaultGear == 1]
  (junction 12) -> Park [order 1] : [DefaultGear == 0]
  (junction 12) -> Park [order 4] : %fallback to park
  drive -> Park [order 2] : [gear_cmd == 0 && allowShift(vc,Tbrake)]
  Park -> Reverse [order 2] : [gear_cmd == -1 && allowShift(vc,Tbrake)]
  Park -> drive [order 1] : [gear_cmd == 1 && allowShift(vc,Tbrake)]
  Reverse -> Park [order 2] : [gear_cmd == 0 && allowShift(vc,Tbrake)]
  drive -> Reverse [order 1] : [gear_cmd == -1 && allowShift(vc,Tbrake)]
  Reverse -> drive [order 1] : [gear_cmd == 1 && allowShift(vc,Tbrake)]
  data: Tdead parameter; Vdead parameter; vel function_input; brakeT function_input; allow function_output; CurrGear output; Tbrake input; vc input; gear_cmd input; DefaultGear parameter
  function allow = allowShift(vel, brakeT):
    | function allow = allowShift(vel, brakeT)
    | allow = (abs(vel) <= Vdead) && (abs(brakeT)>Tdead);
    | end

== matlab function vehicle_hostmodel_2022b_Vignesh/Vehicle Dynamics/VehicleDynamics/engine-steer-brake dynamics/compute net torque ==
  data: gear input; Tnet output; Tengine input; Tbrake input; vc input
function Tnet  = net_torque(gear,Tengine,Tbrake,vc)

%  --set engine torque based on current gear selection

if (gear == 0)
    %  --vehicle is in PARK, so force engine torque to zero
    Tengine = 0;
end

Tnet = Tengine + Tbrake*tanh(5*vc);

end

== matlab function vehicle_hostmodel_2022b_Vignesh/Vehicle Dynamics/VehicleDynamics/engine-steer-brake dynamics/gear selection state machine ==
  data: gear output; gear_cmd input; vc input; Tbrake input; Tdead input; Vdead input
function gear = gear_change_FSM(gear_cmd,vc,Tbrake,Tdead,Vdead)

persistent GEAR

%  The vehicle gear can take on one of the following enumerated values:
%  -1 = REVERSE
%   0 = PARK
%   1 = DRIVE

%  --initialize the local persistent variables

if isempty(GEAR)
    %  --default gear at startup is PARK
    %  Note:  Change this to 1 if you want car to initialize in DRIVE
    GEAR = 0;
end


%  --evaluate the gear change finite state machine

switch GEAR
    case 0  % vehicle is in PARK
        if (gear_cmd == 1)
            %  --check to see if we can shift to DRIVE
            if ((abs(vc) <= Vdead) && (abs(Tbrake) > Tdead))
                %  --shift to DRIVE
                GEAR = 1;
            end
            
        elseif (gear_cmd == 2)
            %  --check to see if we can shift to REVERSE
            if ((abs(vc) <= Vdead) && (abs(Tbrake) > Tdead))
                %  --shift to REVERSE
                GEAR = 2;
            end
        end
        
    case 1  % vehicle is in DRIVE
        if (gear_cmd == 0)
            %  --check to see if we can shift to PARK
            if ((abs(vc) <= Vdead) && (abs(Tbrake) > Tdead))
                %  --shift to PARK
                GEAR = 0;
            end
            
        elseif (gear_cmd == 2)
            %  --check to see if we can shift to REVERSE
            if ((abs(vc) <= Vdead) && (abs(Tbrake) > Tdead))
                %  --shift to REVERSE
                GEAR = 2;
            end
        end
        
    case -1  % vehicle is in REVERSE
        if (gear_cmd == 0)
            %  --check to see if we can shift to PARK
            if ((abs(vc) <= Vdead) && (abs(Tbrake) > Tdead))
                %  --shift to PARK
                GEAR = 0;
            end
            
        elseif (gear_cmd == 1)
            %  --check to see if we can shift to DRIVE
            if ((abs(vc) <= Vdead) && (abs(Tbrake) > Tdead))
                %  --shift to DRIVE
                GEAR = 1;
            end
        end
        
    otherwise  %  --should never be here
        if (vc > Vdead)
            %  --moving forward, so must be in DRIVE
            GEAR = 1;
        elseif (vc < -Vdead)
            %  --moving backward, so must be in REVERSE
            GEAR = 2;
        else
            %  --vehicle stoppped, so must be in PARK
            GEAR = 0;
        end

end


%  --output the current actual gear setting

gear = GEAR;

return

== matlab function vehicle_hostmodel_2022b_Vignesh/Controllers/Lateral Controllers1/Swicth 1 ==
  data: stan input; y output; pure input
function y = fcn(stan, pure)

if stan<pure
    y=stan
else
    y=pure
end

== matlab function vehicle_hostmodel_2022b_Vignesh/Roadrunner Port/Pack Actor Pose/Pose Generation ==
  data: pose input; currPose output
function currPose = generatePose(pose)

yaw = deg2rad(pose(3));
rotm = eul2rotm([yaw 0 0]);

currPose = [[rotm [pose(1:2) 0]']; [0 0 0 1]];

== matlab function vehicle_hostmodel_2022b_Vignesh/Controllers/Lateral Controllers1/Average ==
  data: stan input; y output; pure input
function y = fcn(stan, pure)

y=(stan+pure)/2

== matlab function vehicle_hostmodel_2022b_Vignesh/Subsystem/Function-Call Subsystem/MATLAB Function1 ==
  data: EgoPosition input; MIOPos input; curvature input; MIOVel input; V_i input; xd output; yd output; laneL input; laneR input; V_desired input; LCinProgress output
function [xd,yd,LCinProgress] = traj(EgoPosition,MIOPos,curvature,MIOVel, V_i, laneL, laneR, V_desired)
Vx_i =0;Vx_f=0;Vy_i=0;Vy_f=0;Ax_i=0;Ax_f=0;Ay_i=0;Ay_f=0;T_i=0;T_f=0;V_f=0;A_f=0;x_set=0;y_set=0;theta4=0;

P = zeros(6,6);
% xq = zeros(1,size(RefPath,1)); yq = zeros(1,size(RefPath,2));
EgoPosition(1,2)=-EgoPosition(1,2);
x_init= EgoPosition(1,1)+2; y_init = EgoPosition(1,2)-2;
% xq = RefPath(:,1)'; 
% yq = RefPath(:,2)';
num_foc_t = 98;
V_max= V_desired; ad_n=0; vd_n=MIOVel; wd_n=vd_n*curvature;
lane_width = 3.6 * (laneL-laneR); % +1 if left of current lane and -1 if right of current lane(rahul flipped)
xd = zeros(num_foc_t+1,1); 
yd = zeros(num_foc_t+1,1);
xf =0; 
yf = 0;

    %xf = [EgoPosition(1,1)+ MIOPos(1) ]; yf = [ EgoPosition(1,2)+ MIOPos(2) + lane_width];  
    xf = [EgoPosition(1,1)+ 20 ]; yf = [EgoPosition(1,2)+ lane_width]; % 80
    V_f = V_max;
    W_f = V_f*curvature;
    A_f = 0;

    %dist2crash = sqrt((x_init-MIOPos(1))^2+(y_init-MIOPos(2))^2);
    %dist2crash = 40;
    %T_f = abs(dist2crash/(MIOVel-V_i));
    T_f = 3;
    P = [1, T_i, T_i^2, T_i^3, T_i^4, T_i^5;
         0, 1, 2*T_i, 3*T_i^2, 4*T_i^3, 5*T_i^4;
         0, 0, 2, 6*T_i, 12*T_i^2, 20*T_i^3;
         1, T_f, T_f^2, T_f^3, T_f^4, T_f^5;
         0, 1, 2*T_f, 3*T_f^2, 4*T_f^3, 5*T_f^4;
         0, 0, 2, 6*T_f, 12*T_f^2, 20*T_f^3];

%     mtang4 = (yq(1,index+2)-yq(1,index+1))/(xq(1,index+2)-xq(1,index+1));

    Vx_i = vd_n*cos(theta4); 
    Vy_i = vd_n*sin(theta4); 
    Ax_i = ad_n*cos(theta4)-vd_n*sin(theta4)*wd_n; 
    Ay_i = ad_n*sin(theta4)+vd_n*cos(theta4)*wd_n;

%     if(xq(index+2)-xq(index+1)<0)
%         theta_4 = pi + atan(mtang4);
%     else
%         theta_4 = atan(mtang4);
%     end

    theta_4 =0;
    Vx_f = V_f*cos(theta_4); % curvature angle
    Vy_f = V_f*sin(theta_4);
    Ax_f = A_f*cos(theta_4)-V_f*sin(theta_4)*W_f;
    Ay_f = A_f*sin(theta_4)+V_f*cos(theta_4)*W_f;

    g1 = [x_init; Vx_i; Ax_i; xf; Vx_f; Ax_f];
    g2 = [y_init; Vy_i; Ay_i; yf; Vy_f; Ay_f];

    a_coeff = P\g1;
    b_coeff = P\g2;
    
    td = T_i;
    scatter(x_init,y_init,'go')
    hold on; 
    scatter(xf,yf,'ro')
    hold on;
    
    for f = 1:(num_foc_t+1)
        xd(f,1) = [1,td,td^2,td^3,td^4,td^5]*a_coeff 
        yd(f,1) = [1,td,td^2,td^3,td^4,td^5]*b_coeff
        td = td + (T_f - T_i)/num_foc_t;
        scatter(xd(f,1),yd(f,1),'y.');
    end

LCinProgress = 1;

% hold on;
end

== matlab function vehicle_hostmodel_2022b_Vignesh/Roadrunner Port/Pack Actor Pose/Velocity XYZ Components ==
  data: yaw input size=1; velocity output size=[1 3]; speed input size=1
function velocity = computeVelocity(yaw, speed)

% Output velocity vector (x,y,z)
velocity = speed * [-sind(yaw) cosd(yaw) 0];

== matlab function vehicle_hostmodel_2022b_Vignesh/Roadrunner Port/ENU to NWD/MATLAB Function ==
  data: traj input; destination_traj output; last_idx output
function [destination_traj,last_idx] = DestinationPoint(traj)

last_idx = 1;

for i=1:length(traj)
    if norm(traj(i,1:2)) == 0
        last_idx = i-1;
        break
    end
end

destination_traj = traj(last_idx,1:2);

end

== matlab function vehicle_hostmodel_2022b_Vignesh/Subsystem/Turns LC in prog off ==
  data: u input; y output
function y = fcn(u)

persistent counter;
persistent input_high;

if isempty(counter)
    counter = 0;
end

if isempty(input_high)
    input_high = false;
end

if u ~= 0
    input_high = true;
end

if input_high && counter < 100
    y = u;
    counter = counter + 1;
else
    y = 0;
end

== matlab function vehicle_hostmodel_2022b_Vignesh/Controllers/Lateral Controllers/Subsystem1/MATLAB Function3 ==
  data: velocity input; L_tune output; L_min input; L_max input; velocity_gain input; error_gain input; lateral_error input
function L_tune = fcn(velocity,L_min,L_max,velocity_gain,error_gain,lateral_error)

    if velocity<=5
        L_tune = L_min;
    elseif velocity >5 && velocity<15
        L_chk = abs(velocity_gain*abs(velocity)-error_gain*lateral_error);
        if L_chk < L_min
            L_tune = L_min
        else
            L_tune = L_chk
        end
    else
        L_tune = abs(L_max-error_gain*lateral_error);
    end

== matlab function vehicle_hostmodel_2022b_Vignesh/Controllers/Lateral Controllers/Subsystem1/MATLAB Function4 ==
  settings: updateMethod=DISCRETE
  data: K_out output; current_ref output; r output; theta_p output; cross_track_error output; old_index output; current_error_chk output; lookahead_distance input; pose input; waypoints input; D_sat input; old_index input; new_wp output
function [K_out,current_ref,r,theta_p,cross_track_error,old_index,current_error_chk,new_wp] = fcn(lookahead_distance,pose,waypoints,D_sat,old_index)
    min_ = inf;
    current_ref = zeros(1,2);

    idx = 0;
    id = old_index;

    for j=1:length(waypoints)
        if norm(pose(1:2)-waypoints(j,1:2))<min_
           min_ = norm(pose(1:2)-waypoints(j,1:2));
           current_ref = waypoints(j,1:2);
           idx = j;
           end
    end
    
    old_index = idx;

    new_wp = zeros(1,2);

    flagk = 0;

    for k=idx:length(waypoints)
        if norm(current_ref-waypoints(k,1:2)) > lookahead_distance
            new_wp = waypoints(k,:);
            flagk = 1;
            break  
        end
    end

    if flagk == 0
        min_l = inf;
        new_index = 0
        for l = length(waypoints):-1:(idx+1)
            if norm(current_ref-waypoints(l,1:2))<=min_l
                min_l = norm(current_ref-waypoints(l,1:2));
                new_index = l;
            end
        end
        new_wp = waypoints(l,1:2);
    end 
    
    theta_p = atan2d((new_wp(1,2)-current_ref(1,2)),(new_wp(1,1)-current_ref(1,1)));

    current_heading = pose(1,3);

    lookahead_angle = (theta_p-current_heading);

    d_new = 0;
    d_calc = 0;

    A = [cosd(theta_p+pi/2) -cosd(current_heading+lookahead_angle);sind(theta_p+pi/2) -sind(current_heading+lookahead_angle)];

    vec_dif = current_ref-new_wp;

    new_vec = zeros(2,1);

    if det(A)>1e-5
        new_vec = A\vec_dif';
        d_calc = new_vec(1,1);
        if d_calc>=D_sat
            d_new = sign(d_calc)*D_sat;
        else
            d_new = d_calc;
        end

        wp_sel = new_wp - [d_new*cosd(theta_p+pi/2) d_new*sind(theta_p+pi/2)];
    else
        wp_sel = new_wp;
    end

    vec_car_frame = [cosd(current_heading) sind(current_heading);-sind(current_heading) cosd(current_heading)]*(wp_sel'-current_ref');

    r = lookahead_distance^2/(2*vec_car_frame(2,1));

    K_out = 1/r;

  
    %{
    if abs(old_curvature) < 0.01 & abs(K_computed) < 0.01
        K_out = 0;
    else
        K_out = K_computed;
    end
    %}
    
   


    K_ref = 2*sind(lookahead_angle)/lookahead_distance;
    

    
    cross_track_error = vec_car_frame(2,1);

    computed_error =  norm(current_ref'-pose(1:2)');

  
    if computed_error<0.01
        current_error_chk = 0;
    else
        current_error_chk = computed_error;
    end

== matlab function vehicle_hostmodel_2022b_Vignesh/Controllers/Lateral Controllers/Subsystem1/MATLAB Function5 ==
  data: error_la output; Lad input; theta_p input; pose input; cross_track_error input; L input
function error_la = fcn(Lad,theta_p,pose,cross_track_error,L)
    current_angle = pose(3);
    heading_error = theta_p-current_angle;
    error_la = cross_track_error+(L/2+Lad)*sind(heading_error);

== matlab function vehicle_hostmodel_2022b_Vignesh/Controllers/Lateral Controllers/Subsystem1/MATLAB Function6 ==
  data: r input; theta output; L input
function theta = fcn(r,L)

theta = atan(L/r);

== matlab function vehicle_hostmodel_2022b_Vignesh/Subsystem/PathPlanner/MATLAB Function3 ==
  settings: updateMethod=DISCRETE
  data: out output; check output; Xref input; Yref input; xd input; yd input; LC input; current_pos input; d2f input; dcheck output
function [out,check,dcheck]  = PathPlanning(Xref, Yref, xd, yd, LC, current_pos, d2f)

persistent output_matrix
persistent lc_triggered

if isempty(lc_triggered)
lc_triggered = false;
end

%lc_triggered=0;
%if isempty(hold_output)
  %  hold_output = false;
%end


if isempty(output_matrix)
    output_matrix = [Xref(:), Yref(:)];
    out = [Xref(:), Yref(:)];
else
    out = output_matrix;
end

if LC && ~isempty(xd) && ~isempty(yd)
    output_matrix = [xd(:), yd(:)];
    lc_triggered=true;
       
end

check=lc_triggered;
dcheck=output_matrix;
%out=output_matrix;

if lc_triggered && d2f < 5 %&& ~isempty(output_matrix) %&& ~hold_output
    %Yout = Yref(:);
    if current_pos > 0
        Xout = Xref(:);
        Yout = Yref + 3.6;
    else
        Xout = Xref(:);
        Yout = Yref;
    end
    output_matrix = [Xout, Yout];
    out=output_matrix;
    lc_triggered=false;
    %hold_output = true;
end

out=output_matrix;




%if ~LC && ~isempty(output_matrix) && lc_triggered
    %hold_output = false;
    %lc_triggered=false;
%end

end

== matlab function vehicle_hostmodel_2022b_Vignesh/Roadrunner Port/ENU to NWD/MATLAB Function1 ==
  data: traj input; trajectory_way output
function trajectory_way = fcn(traj)

last_idx = 1;

for i=1:length(traj)
    if norm(traj(i,1:2)) == 0
        last_idx = i-1;
        break
    end
end

trajectory_way = zeros(150,2);

for j = 1:last_idx
    trajectory_way(j,:) = traj(j,1:2);
end


for k = (last_idx+1):100
    trajectory_way(k,:) = trajectory_way(last_idx,:);
end
